simulink model "EarlyReturn13_2018a"  (R2018a)
settings: Solver=VariableStepAuto  StartTime=0.0  StopTime=0.1  RelTol=1e-3
settings Model: Creator=BEAR  LastModifiedBy=bzhan

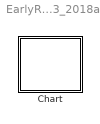
== system EarlyReturn13_2018a ==
  Chart : Stateflow chart  TreatAsAtomicUnit=on

== stateflow chart EarlyReturn13_2018a/Chart ==
  state A [parallel]
    settings: executionOrder=1
    state A1
      ex: f("exA1");
      x=x-1;E;
      f("exA1_done")
    state A2
      en: f("enA2")
    state A3
      en: f("enA3")
    (default) -> A1 : {x=5;}
    A1 -> A2 [order 2] : F
    A1 -> A3 [order 1] : E[x>0]
  state B [parallel]
    settings: executionOrder=2
    state B1
    state B2
    (default) -> B1
    B1 -> B2 : /{f("F");F}
  data: s function_input; x local
  events: E local FUNCTION_CALL_EVENT; F local FUNCTION_CALL_EVENT
  function f(s):
    | function f(s)
    |   fprintf(s+"\n");
